simulink model "sim_SysContinu"  (R2020a)
settings: Solver=VariableStepAuto  StartTime=0.0  StopTime=20e-3  RelTol=1e-3
values from neighbouring files (symbols this model uses):
  Kp = 1    [SysContinu.m]
  Taum = Lm/Rm    (= 0.002)    [BE Trotinette.m]    (also in SysContinu.m)
  Te = 2e-4    (= 0.0002)    [BE Trotinette.m]    (also in SysContinu.m)
  Ubat = 24    [BE Trotinette.m]    (also in SysContinu.m)
settings Model: Creator=bouzerga  LastModifiedBy=kttran

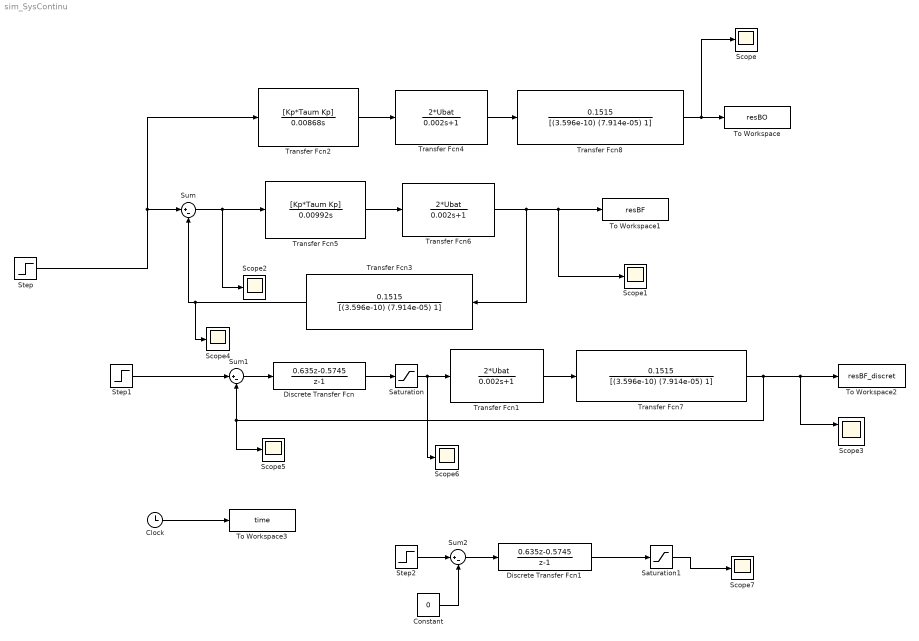
== system sim_SysContinu ==
  Clock : Clock
  Constant : Constant  Value=0
  Discrete Transfer Fcn : DiscreteTransferFcn  Numerator=[0.635 -0.5745]  Denominator=[1 -1]  SampleTime=Te
  Discrete Transfer Fcn1 : DiscreteTransferFcn  Numerator=[0.635 -0.5745]  Denominator=[1 -1]  SampleTime=Te
  Saturation : Saturate
  Saturation1 : Saturate
  Scope{,1..2,4..7} (7 alike) : Scope
  Scope3 : Scope  NumInputPorts=2
  Step : Step  Time=5e-3  Before=-0.1  After=0.1  SampleTime=0
  Step1 : Step  Time=0.1  After=0.5  SampleTime=0
  Step2 : Step  Time=0.1  After=0.1  SampleTime=0
  Sum : Sum  Inputs=|+-
  Sum1 : Sum  Inputs=|+-
  Sum2 : Sum  Inputs=|+-
  To Workspace : ToWorkspace  VariableName=resBO  SaveFormat=Timeseries  SampleTime=-1
  To Workspace1 : ToWorkspace  VariableName=resBF  SaveFormat=Timeseries  SampleTime=-1
  To Workspace2 : ToWorkspace  VariableName=resBF_discret  SaveFormat=Timeseries  SampleTime=-1
  To Workspace3 : ToWorkspace  VariableName=time  SaveFormat=Timeseries  SampleTime=-1
  Transfer Fcn1 : TransferFcn  Numerator=2*Ubat  Denominator=[0.002 1]
  Transfer Fcn2 : TransferFcn  Numerator=[Kp*Taum Kp]  Denominator=[0.00868 0]
  Transfer Fcn3 : TransferFcn  Numerator=0.1515  Denominator=[(3.596e-10) (7.914e-05) 1]
  Transfer Fcn4 : TransferFcn  Numerator=2*Ubat  Denominator=[0.002 1]
  Transfer Fcn5 : TransferFcn  Numerator=[Kp*Taum Kp]  Denominator=[0.00992 0]
  Transfer Fcn6 : TransferFcn  Numerator=2*Ubat  Denominator=[0.002 1]
  Transfer Fcn7 : TransferFcn  Numerator=0.1515  Denominator=[(3.596e-10) (7.914e-05) 1]
  Transfer Fcn8 : TransferFcn  Numerator=0.1515  Denominator=[(3.596e-10) (7.914e-05) 1]
  wires:
  Step/1 -> Transfer Fcn2/1, Sum/1
  Transfer Fcn6/1 -> Scope1/1, To Workspace1/1, Transfer Fcn3/1
  Sum/1 -> Scope2/1, Transfer Fcn5/1
  Transfer Fcn5/1 -> Transfer Fcn6/1
  Transfer Fcn3/1 -> Scope4/1, Sum/2
  Sum1/1 -> Discrete Transfer Fcn/1
  Transfer Fcn1/1 -> Transfer Fcn7/1
  Transfer Fcn7/1 -> Scope3/1, To Workspace2/1, Sum1/2, Scope5/1
  Clock/1 -> To Workspace3/1
  Transfer Fcn8/1 -> Scope/1, To Workspace/1
  Transfer Fcn4/1 -> Transfer Fcn8/1
  Transfer Fcn2/1 -> Transfer Fcn4/1
  Step1/1 -> Sum1/1
  Discrete Transfer Fcn/1 -> Saturation/1
  Saturation/1 -> Scope6/1, Transfer Fcn1/1
  Step2/1 -> Sum2/1
  Sum2/1 -> Discrete Transfer Fcn1/1
  Discrete Transfer Fcn1/1 -> Saturation1/1
  Saturation1/1 -> Scope7/1
  Constant/1 -> Sum2/2
